simulink model "frbd_64ch_600mhz"  (R2013b)
settings: Solver=FixedStepDiscrete  SolverMode=SingleTasking  StartTime=0.0  StopTime=10.0  RelTol=1e-3
undefined symbols (not defined in the file or in its folder): pfb_coeff_gen_calc
libraries: xbsIndex_r4 x14695, casper_library_misc x59, casper_library_delays x32, dspsigops x16, casper_library_pfbs x2, xps_library x1
(part 9 of 145)

== system frbd_64ch_600mhz/frb_detector9 ==
  out_reg : Inport
  assert_reg : xbsIndex_r4/Assert  assert_type=on  type_source=Explicitly  gui_display_data_type=Boolean  arith_type=Boolean  n_bits=32  bin_pt=0  preci_type=Single  exp_width=8  frac_width=24  assert_rate=off  rate_source=Explicitly  period=1  output_port=on  block_type=assert
  cast_gw : xbsIndex_r4/Convert  gui_display_data_type=Fixed-point  arith_type=Unsigned  n_bits=32  bin_pt=0  float_type=Single  exp_bits=8  fraction_bits=24  quantization=Truncate  overflow=Wrap  en=off  latency=0  dbl_ovrd=off  pipeline=off  block_type=convert
  frbd_64ch_600mhz2_frb_detector9_user_data_in : xbsIndex_r4/Gateway Out  inherit_from_input=off  hdl_port=on  timing_constraint=None  locs_specified=off  LOCs={}  UseAsDAC=off  DACChannel='1'  block_type=gatewayout
  io_delay : xbsIndex_r4/Delay  rst=off  infoeditControl=Selection of Reset will increase slice count due to use of real FFs and instead of SRLs  en=off  latency=0  dbl_ovrd=off  reg_retiming=on  block_type=delay
  reint1 : xbsIndex_r4/Reinterpret  force_arith_type=on  arith_type=Unsigned  force_bin_pt=on  bin_pt=0  block_type=reinterpret
  sim_out : Terminator
  wires:
  io_delay/1 -> cast_gw/1
  cast_gw/1 -> frbd_64ch_600mhz2_frb_detector9_user_data_in/1
  frbd_64ch_600mhz2_frb_detector9_user_data_in/1 -> sim_out/1
  out_reg/1 -> assert_reg/1
  assert_reg/1 -> reint1/1
  reint1/1 -> io_delay/1

== system frbd_64ch_600mhz/gain ==
  sim_1 : Inport
  frbd_64ch_600mhz2_gain_user_data_out : xbsIndex_r4/Gateway In  gui_display_data_type=Fixed-point  arith_type=Unsigned  n_bits=32  bin_pt=0  preci_type=Single  exp_width=8  frac_width=24  quantization="Round  (unbiased: +/- Inf)"  overflow=Saturate  period=1  dbl_ovrd=off  timing_constraint=None  locs_specified=off  LOCs={}  UseAsADC=off  ADCChannel='1'  inherit_from_input=off  hdl_port=on  block_type=gatewayin
  io_delay : xbsIndex_r4/Delay  rst=off  infoeditControl=Selection of Reset will increase slice count due to use of real FFs and instead of SRLs  en=off  latency=0  dbl_ovrd=off  reg_retiming=on  block_type=delay
  reint1 : xbsIndex_r4/Reinterpret  force_arith_type=on  arith_type=Unsigned  force_bin_pt=on  bin_pt=0  block_type=reinterpret
  slice_reg : xbsIndex_r4/Slice  nbits=32  boolean_output=off  mode=Lower Bit Location + Width  bit1=0  base1=MSB of Input  bit0=0  base0=LSB of Input  dbl_ovrd=off  block_type=slice
  in_reg : Outport
  wires:
  frbd_64ch_600mhz2_gain_user_data_out/1 -> io_delay/1
  sim_1/1 -> frbd_64ch_600mhz2_gain_user_data_out/1
  io_delay/1 -> slice_reg/1
  slice_reg/1 -> reint1/1
  reint1/1 -> in_reg/1

== system frbd_64ch_600mhz/m0_tree ==
  In1 : Inport
  delay_tree : Subsystem  AncestorBlock=casper_library_delays/delay_tree  mask(delay_tree){fanout=12, bfac=2}
      mask prompts: bfac "Branching factor"
      mask help: A tree of delays.
      mask init:
      | delay_tree_init(gcb, ...
      |     'fanout', fanout, ...
      |     'bfac', bfac);
      settings: AttributesFormatString=delay=5
  tag scope: m0d0=global, m0d10=global, m0d11=global, m0d1=global, m0d2=global, m0d3=global, m0d4=global, m0d5=global, m0d6=global, m0d7=global, m0d8=global, m0d9=global
  wires:
  delay_tree/4(out4) -> [m0d3]
  delay_tree/9(out9) -> [m0d8]
  In1/1 -> delay_tree/1(in)
  delay_tree/5(out5) -> [m0d4]
  delay_tree/8(out8) -> [m0d7]
  delay_tree/7(out7) -> [m0d6]
  delay_tree/10(out10) -> [m0d9]
  delay_tree/12(out12) -> [m0d11]
  delay_tree/6(out6) -> [m0d5]
  delay_tree/2(out2) -> [m0d1]
  delay_tree/3(out3) -> [m0d2]
  delay_tree/1(out1) -> [m0d0]
  delay_tree/11(out11) -> [m0d10]

== system frbd_64ch_600mhz/m1_tree ==
  In1 : Inport
  delay_tree : Subsystem  AncestorBlock=casper_library_delays/delay_tree  mask(delay_tree){fanout=12, bfac=2}
      mask prompts: bfac "Branching factor"
      mask help: A tree of delays.
      mask init:
      | delay_tree_init(gcb, ...
      |     'fanout', fanout, ...
      |     'bfac', bfac);
      settings: AttributesFormatString=delay=5
  tag scope: m1d0=global, m1d10=global, m1d11=global, m1d1=global, m1d2=global, m1d3=global, m1d4=global, m1d5=global, m1d6=global, m1d7=global, m1d8=global, m1d9=global
  wires:
  delay_tree/11(out11) -> [m1d10]
  delay_tree/1(out1) -> [m1d0]
  delay_tree/3(out3) -> [m1d2]
  delay_tree/2(out2) -> [m1d1]
  delay_tree/6(out6) -> [m1d5]
  delay_tree/12(out12) -> [m1d11]
  delay_tree/10(out10) -> [m1d9]
  delay_tree/7(out7) -> [m1d6]
  delay_tree/8(out8) -> [m1d7]
  delay_tree/5(out5) -> [m1d4]
  In1/1 -> delay_tree/1(in)
  delay_tree/9(out9) -> [m1d8]
  delay_tree/4(out4) -> [m1d3]

== system frbd_64ch_600mhz/m2_tree ==
  In1 : Inport
  delay_tree : Subsystem  AncestorBlock=casper_library_delays/delay_tree  mask(delay_tree){fanout=12, bfac=2}
      mask prompts: bfac "Branching factor"
      mask help: A tree of delays.
      mask init:
      | delay_tree_init(gcb, ...
      |     'fanout', fanout, ...
      |     'bfac', bfac);
      settings: AttributesFormatString=delay=5
  tag scope: m2d0=global, m2d10=global, m2d11=global, m2d1=global, m2d2=global, m2d3=global, m2d4=global, m2d5=global, m2d6=global, m2d7=global, m2d8=global, m2d9=global
  wires:
  delay_tree/4(out4) -> [m2d3]
  delay_tree/9(out9) -> [m2d8]
  In1/1 -> delay_tree/1(in)
  delay_tree/5(out5) -> [m2d4]
  delay_tree/8(out8) -> [m2d7]
  delay_tree/7(out7) -> [m2d6]
  delay_tree/10(out10) -> [m2d9]
  delay_tree/12(out12) -> [m2d11]
  delay_tree/6(out6) -> [m2d5]
  delay_tree/2(out2) -> [m2d1]
  delay_tree/3(out3) -> [m2d2]
  delay_tree/1(out1) -> [m2d0]
  delay_tree/11(out11) -> [m2d10]

== system frbd_64ch_600mhz/m3_tree ==
  In1 : Inport
  delay_tree : Subsystem  AncestorBlock=casper_library_delays/delay_tree  mask(delay_tree){fanout=12, bfac=2}
      mask prompts: bfac "Branching factor"
      mask help: A tree of delays.
      mask init:
      | delay_tree_init(gcb, ...
      |     'fanout', fanout, ...
      |     'bfac', bfac);
      settings: AttributesFormatString=delay=5
  tag scope: m3d0=global, m3d10=global, m3d11=global, m3d1=global, m3d2=global, m3d3=global, m3d4=global, m3d5=global, m3d6=global, m3d7=global, m3d8=global, m3d9=global
  wires:
  delay_tree/11(out11) -> [m3d10]
  delay_tree/1(out1) -> [m3d0]
  delay_tree/3(out3) -> [m3d2]
  delay_tree/2(out2) -> [m3d1]
  delay_tree/6(out6) -> [m3d5]
  delay_tree/12(out12) -> [m3d11]
  delay_tree/10(out10) -> [m3d9]
  delay_tree/7(out7) -> [m3d6]
  delay_tree/8(out8) -> [m3d7]
  delay_tree/5(out5) -> [m3d4]
  In1/1 -> delay_tree/1(in)
  delay_tree/9(out9) -> [m3d8]
  delay_tree/4(out4) -> [m3d3]
